simulink library "rappid_564xl_ec_toolbox"  (Simulink 8.1)
settings: Solver=FixedStepDiscrete  StartTime=0.0  StopTime=10.0  RelTol=1e-3
undefined symbols (not defined in the file or in its folder): CTU_unit, mem_AddrLW, mem_AddrUP, rappid_564xl_adc_input_support_rev2, rappid_564xl_can_support_rev2, read_mem_AddrLW, read_mem_AddrUP
(part 2 of 5)

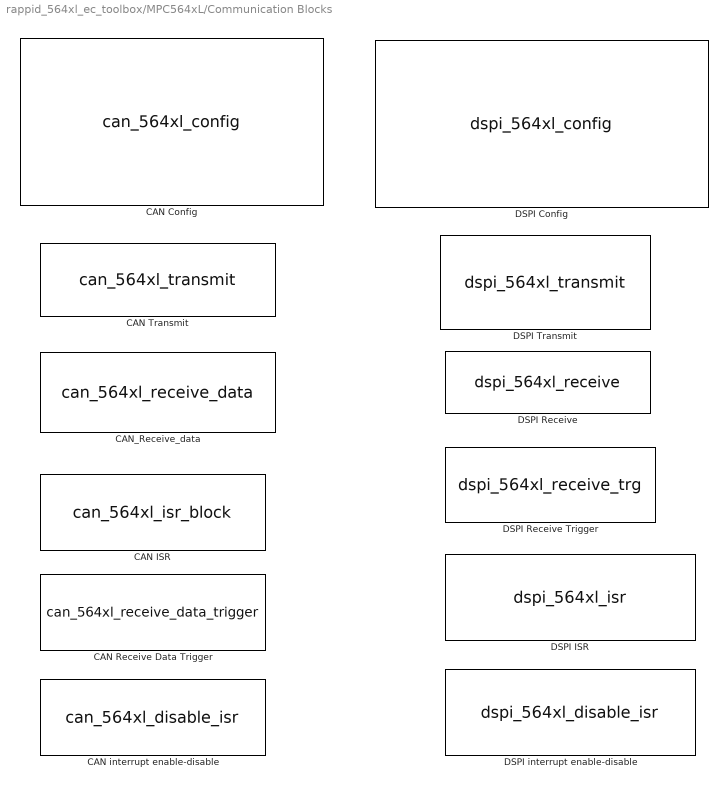
== system rappid_564xl_ec_toolbox/MPC564xL/Communication Blocks ==
  CAN Config : S-Function  Priority=1  LoadFcn=rappid_564xl_can_support_rev2(gcb);  FunctionName=can_564xl_config  Parameters=can_unit_v2, MCR, CTRL  EnableBusSupport=off  mask(flexcan_564xl_config_block){can_unit=A, can_unit_v2=0, can_idam=A - One full ID (standard or extended) per filter element., can_srx_dis=1 - Self reception disabled, can_presdiv=4, can_rjw=3, can_pseg1=3, can_pseg2=3, can_clk_src=0 - The CAN engine clock source is the oscillator clock, can_lpb=0 - Loop Back disabled, can_smp=1 - Three samples are used to determine the value of the received bit, can_boff_rec=0 - Automatic recovering from Bus Off state enabled, can_tsyn=0 - Timer Sync feature disabled, can_lbuf=0 - Buffer with highest priority is transmitted first, can_lom=0 - Listen Only Mode is deactivated, can_propseg=6}
      mask prompts: can_unit "CAN Bus"; can_unit_v2 "CAN Bus"; can_idam "ID Acceptance Mode"; can_srx_dis "Self Reception Disable"; can_presdiv "Prescaler Divider (0-255)"; can_rjw "Resync Jump Width"; can_pseg1 "Phase Segment 1"; can_pseg2 "Phase Segment 2"; can_clk_src "CAN Engine Clock Source"; can_lpb "Loop Back"; can_smp "Sampling Mode"; can_boff_rec "Bus Off Recovery Mode"; can_tsyn "Timer Sync Mode"; can_lbuf "Lowest Buffer Transmitted First"; can_lom "Listen-Only Mode"; can_propseg "Propagation Segment"
      mask help: This block allows to configure the FlexCan module.
      mask init:
      | crlf = sprintf('\n');
      | 
      | canUnit     = num2str(get_param(gcb,'can_unit_v2'));
      | canIDAM     = get_param(gcb,'can_idam');
      | 
      | MCR = 1342177343;
      | if (strcmp(canIDAM,'A - One full ID (standard or extended) per filter element.'))
      |     canIDAM = 'A - One full ID ';
      | elseif (strcmp(canIDAM,'B - Two full standard IDs or two partial 14-bit extended IDs per filter element.'))
      |     canIDAM = 'B - Two full standard IDs';
      |     MCR = bitset(uint32(MCR), 32-23);
      | elseif (strcmp(canIDAM,'C - Four partial 8-bit IDs (standard or extended) per filter element.'))
      |     canIDAM = 'C - Four partial 8-bit IDs';
      |     MCR = bitset(uint32(MCR), 32-22);
      | elseif (strcmp(canIDAM,'D - All frames rejected.'))
      |     canIDAM = 'Rejected';
      |     MCR = bitset(uint32(MCR), 32-23);
      |     MCR = bitset(uint32(MCR), 32-22);
      | end
      | 
      | if ( strcmp( num2str(get_param(gcb,'can_srx_dis')), 'on'))
      |     MCR = bitset(uint32(MCR), 32-14);
      | end
      | 
      | CTRL = 0;
      | 
      | CTRL = bitshift(uint32(str2num(get_param(gcb, 'can_presdiv'))),31-7);
      | CTRL = bitor( CTRL, bitshift(uint32(str2num(get_param(gcb, 'can_rjw'))),31-9));
      | CTRL = bitor( CTRL, bitshift(uint32(str2num(get_param(gcb, 'can_pseg1'))),31-12));
      | CTRL = bitor( CTRL, bitshift(uint32(str2num(get_param(gcb, 'can_pseg2'))),31-15));
      | 
      | if ( strcmp( get_param(gcb,'can_clk_src'), '1 - The CAN engine clock source is the bus clock'))
      |     CTRL = bitset(uint32(CTRL), 32-18);
      | end
      | 
      | if ( strcmp( get_param(gcb,'can_lpb'), '1 - Loop Back enabled'))
      |     CTRL = bitset(uint32(CTRL), 32-19);
      | end
      | 
      | if ( strcmp( get_param(gcb,'can_smp'), '1 - Three samples are used to determine the value of the received bit'))
      |     CTRL = bitset(uint32(CTRL), 32-24);
      | end
      | 
      | if ( strcmp( get_param(gcb,'can_boff_rec'), '1 - Automatic recovering from Bus Off state disabled'))
      |     CTRL = bitset(uint32(CTRL), 32-25);
      | end
      | 
      | if ( strcmp( get_param(gcb,'can_tsyn'), '1 - Timer Sync feature enabled'))
      |     CTRL = bitset(uint32(CTRL), 32-26);
      | end
      | 
      | if ( strcmp( get_param(gcb,'can_lbuf'), '1 - Lowest number buffer is transmitted first'))
      |     CTRL = bitset(uint32(CTRL), 32-27);
      | end
      | 
      | if ( strcmp( get_param(gcb,'can_lom'), '1 - FlexCAN module operates in Listen Only Mode'))
      |     CTRL = bitset(uint32(CTRL), 32-28);
      | end
      | 
      | CTRL = bitor( CTRL, bitshift(uint32(str2num(get_param(gcb, 'can_propseg'))),31-31));
      | 
      | maskStr = [ 'CAN Bus ',canUnit, crlf,...
      |     'ID Acceptance Mode ', canIDAM,...
      |     ];
      | 
      | if strcmp(canUnit ,'0')
      |    value_new = 'A';
      | else                                     
      |    value_new = 'B';         
      | end                                                                               
      | set_param(gcb, 'can_unit', value_new);
      mask Help: web([rappid_block_help,filesep,'CAN_config.htm']);
      mask TypeOptions can_unit: A | B
      mask TypeOptions can_unit_v2: 0 | 1
      mask TypeOptions can_idam: A - One full ID (standard or extended) per filter element. | B - Two full standard IDs or two partial 14-bit extended IDs per filter element. | C - Four partial 8-bit IDs (standard or extended) per filter element. | D - All frames rejected.
      mask TypeOptions can_srx_dis: 0 - Self reception enabled | 1 - Self reception disabled
      mask TypeOptions can_rjw: 0 | 1 | 2 | 3
      mask TypeOptions can_pseg1: 0 | 1 | 2 | 3 | 4 | 5 | 6 | 7
      mask TypeOptions can_pseg2: 1 | 2 | 3 | 4 | 5 | 6 | 7
      mask TypeOptions can_clk_src: 0 - The CAN engine clock source is the oscillator clock | 1 - The CAN engine clock source is the bus clock
      mask TypeOptions can_lpb: 0 - Loop Back disabled | 1 - Loop Back enabled
      mask TypeOptions can_smp: 0 - One sample is used to determine the bit value | 1 - Three samples are used to determine the value of the received bit
      mask TypeOptions can_boff_rec: 0 - Automatic recovering from Bus Off state enabled | 1 - Automatic recovering from Bus Off state disabled
      mask TypeOptions can_tsyn: 0 - Timer Sync feature disabled | 1 - Timer Sync feature enabled
      mask TypeOptions can_lbuf: 0 - Buffer with highest priority is transmitted first | 1 - Lowest number buffer is transmitted first
      mask TypeOptions can_lom: 0 - Listen Only Mode is deactivated | 1 - FlexCAN module operates in Listen Only Mode
      mask TypeOptions can_propseg: 0 | 1 | 2 | 3 | 4 | 5 | 6 | 7
      mask Display: disp(maskStr)
  CAN ISR : S-Function  LoadFcn=rappid_564xl_can_support_rev2(gcb);  FunctionName=can_564xl_isr_block  Parameters=can_unit_v2, can_isr_prio, canMode, canFlags  EnableBusSupport=off  mask(flexcan_564xl_isr_block){can_unit=A, can_unit_v2=0, can_isr_prio=1, can_isr_mode=Errors, can_wrn_tx=on, can_wrn_rx=on}
      mask prompts: can_unit "CAN Bus"; can_unit_v2 "CAN Bus"; can_isr_prio "ISR Priority"; can_isr_mode "Can ISR"; can_wrn_tx "Tx Warning Interrupt"; can_wrn_rx "Rx Warning Interrupt"
      mask help: This block allows user to process FlexCan ISR's
      mask init:
      | crlf = sprintf('\n');
      | 
      | canUnit     = num2str(get_param(gcb,'can_unit_v2'));
      | canISRPrio  = num2str(get_param(gcb,'can_isr_prio'));
      | canISRMode  = get_param(gcb, 'can_isr_mode');
      | canTxWrn    = get_param(gcb, 'can_wrn_tx');
      | canRxWrn    = get_param(gcb, 'can_wrn_rx');
      | 
      | canMode = 0;
      | TxWrn = 0;
      | RxWrn = 0;
      | 
      | maskStr = [ 'CAN Bus ',canUnit, crlf, 'ISR Priority ',canISRPrio, crlf,...
      |         'CAN ISR Mode ',canISRMode, crlf];
      |              
      | if (strcmp(canISRMode,'Warnings'))
      |     maskStr = [ maskStr, 'TxWarning ', canTxWrn, crlf, 'RxWarning' canRxWrn];
      |     
      |     canMode = 1;
      |     
      |     if (strcmp(canTxWrn,'on'))
      |         TxWrn = 1;
      |     end
      |     if (strcmp(canRxWrn,'on'))
      |         RxWrn = 1;
      |     end
      |    
      |     
      | end
      | canFlags =[TxWrn, RxWrn]; 
      | 
      | if strcmp(canUnit ,'0')
      |    value_new = 'A';
      | else                                     
      |    value_new = 'B';         
      | end                                                                               
      | set_param(gcb, 'can_unit', value_new);
      mask Help: web([rappid_block_help,filesep,'CAN_isr.htm']);
      mask TypeOptions can_unit: A | B
      mask TypeOptions can_unit_v2: 0 | 1
      mask TypeOptions can_isr_prio: 1 | 2 | 3 | 4 | 5 | 6 | 7 | 8 | 9 | 10 | 11 | 12 | 13 | 14 | 15
      mask TypeOptions can_isr_mode: Errors | Warnings
      mask Callback can_isr_mode:
      | maskVis = get_param(gcb, 'MaskVisibilities');
      | 
      | if (strcmp (get_param(gcb, 'can_isr_mode'), 'Errors'))
      |     maskVis{5} = 'off';
      |     maskVis{6} = 'off';
      | else
      |     maskVis{5} = 'on';
      |     maskVis{6} = 'on';
      | end
      | 
      | set_param(gcb,'MaskVisibilities', maskVis);
      mask Display:
      | disp(maskStr)
      | port_label('output', 1, 'Trigger');
      | port_label('output', 2, 'Mask');
  CAN Receive Data Trigger : S-Function  LoadFcn=rappid_564xl_can_support_rev2(gcb);  FunctionName=can_564xl_receive_data_trigger  Parameters=can_unit_v2, can_buffer, can_id  EnableBusSupport=off  mask(flexcan_564xl_receive_data_trigger_block){can_unit=A, can_unit_v2=0, can_buffer=0, can_id=0, can_isr_prio=0}
      mask prompts: can_unit "CAN Bus"; can_unit_v2 "CAN Bus"; can_buffer "Buffer (0 to 31)"; can_id "ID"; can_isr_prio "ISR Priority"
      mask help: This block allows user to receive data through CAN interface
      mask init:
      | crlf = sprintf('\n');
      | 
      | canUnit     = num2str(get_param(gcb,'can_unit_v2'));
      | canBuffer   = num2str(get_param(gcb,'can_buffer'));
      | canID       = num2str(get_param(gcb,'can_id'));
      | canISRPrio  = num2str(get_param(gcb,'can_isr_prio'));
      | maskStr = [ 'CAN Bus ',canUnit, crlf,'CAN Buffer ', canBuffer, crlf...
      |     'CAN Message ID ', canID, crlf, 'CAN ISR Priority ', canISRPrio ];
      | 
      | if strcmp(canUnit ,'0')
      |    value_new = 'A';
      | else                                     
      |    value_new = 'B';         
      | end                                                                               
      | set_param(gcb, 'can_unit', value_new);
      mask Help: web([rappid_block_help,filesep,'CAN_receive_trigger.htm']);
      mask TypeOptions can_unit: A | B
      mask TypeOptions can_unit_v2: 0 | 1
      mask TypeOptions can_buffer: 0 | 1 | 2 | 3 | 4 | 5 | 6 | 7 | 8 | 9 | 10 | 11 | 12 | 13 | 14 | 15 | 16 | 17 | 18 | 19 | 20 | 21 | 22 | 23 | 24 | 25 | 26 | 27 | 28 | 29 | 30 | 31
      mask TypeOptions can_isr_prio: 0 | 1 | 2 | 3 | 4 | 5 | 6 | 7 | 8 | 9 | 10 | 11 | 12 | 13 | 14 | 15
      mask Display:
      | disp(maskStr)
      | port_label('output', 1, 'Trigger');
      | port_label('output', 2, 'ID');
      | port_label('output', 3, 'ID Type');
      | port_label('output', 4, 'Message');
      | port_label('output', 5, 'Time stamp');
  CAN Transmit : S-Function  LoadFcn=rappid_564xl_can_support_rev2(gcb);  FunctionName=can_564xl_transmit  Parameters=can_unit_v2, can_buffer, can_id  EnableBusSupport=off  mask(flexcan_564xl_transmit_block){can_unit=A, can_unit_v2=0, can_buffer=0, can_id=0}
      mask prompts: can_unit "CAN Bus"; can_unit_v2 "CAN Bus"; can_buffer "Buffer (0 to 31)"; can_id "ID"
      mask help: This block allows user to transmit data throught CAN interface.
      mask init:
      | crlf = sprintf('\n');
      | 
      | canUnit     = num2str(get_param(gcb,'can_unit_v2'));
      | canBuffer   = num2str(get_param(gcb,'can_buffer'));
      | canID       = num2str(get_param(gcb,'can_id'));
      | maskStr = [ 'CAN Bus ',canUnit, crlf,'CAN Buffer ', canBuffer, crlf...
      |     'CAN Message ID ', canID];
      | 
      | if strcmp(canUnit ,'0')
      |    value_new = 'A';
      | else                                     
      |    value_new = 'B';         
      | end                                                                               
      | set_param(gcb, 'can_unit', value_new);
      mask Help: web([rappid_block_help,filesep,'CAN_transmit.htm']);
      mask TypeOptions can_unit: A | B
      mask TypeOptions can_unit_v2: 0 | 1
      mask TypeOptions can_buffer: 0 | 1 | 2 | 3 | 4 | 5 | 6 | 7 | 8 | 9 | 10 | 11 | 12 | 13 | 14 | 15 | 16 | 17 | 18 | 19 | 20 | 21 | 22 | 23 | 24 | 25 | 26 | 27 | 28 | 29 | 30 | 31
      mask Display:
      | disp(maskStr)
      | port_label('input', 1, 'Message');
      | port_label('input', 2, 'Lenght');
  CAN interrupt enable-disable : S-Function  FunctionName=can_564xl_disable_isr  Parameters="can_unit,   canFlags"  EnableBusSupport=off  mask(flexcan_564xl_isr_enable){can_unit=0, can_err_enable=off, can_wrn_tx=off, can_wrn_rx=off}
      mask prompts: can_unit "CAN Bus"; can_err_enable "Enable Error Interrupt"; can_wrn_tx "Enable Tx Warning Interrupt"; can_wrn_rx "Enable Rx Warning Interrupt"
      mask help: This block enables or disables the interrupt for each PIT block.
      mask init:
      | crlf = sprintf('\n');
      | 
      | canUnit     = num2str(get_param(gcb,'can_unit'));
      | canErr      = get_param(gcb, 'can_err_enable');
      | canTxWrn    = get_param(gcb, 'can_wrn_tx');
      | canRxWrn    = get_param(gcb, 'can_wrn_rx');
      | 
      | maskStr = [ 'CAN Bus: ', canUnit, crlf, 'Error interrupt: ', canErr, crlf, 'TX Warning interrupt: ', canTxWrn, crlf,'RX Warning interrupt: ', canRxWrn]; 
      | 
      | ErrInt = 0;
      | TxWrn = 0;
      | RxWrn = 0;
      | 
      | if (strcmp(canTxWrn,'on'))
      |     TxWrn = 1;
      | end
      | if (strcmp(canRxWrn,'on'))
      |     RxWrn = 1;
      | end
      | if (strcmp(canErr,'on'))
      |     ErrInt = 1;
      | end
      |      
      | canFlags =[TxWrn, RxWrn, ErrInt];
      mask Help: web([rappid_block_help,filesep,'CAN_isr_enable.htm']);
      mask TypeOptions can_unit: 0 | 1
      mask Display: disp(maskStr)
  CAN_Receive_data : S-Function  LoadFcn=rappid_564xl_can_support_rev2(gcb);  FunctionName=can_564xl_receive_data  Parameters=can_unit_v2, can_buffer, can_id  EnableBusSupport=off  mask(flexcan_564xl_receive_data_block){can_unit=A, can_unit_v2=0, can_buffer=0, can_id=0}
      mask prompts: can_unit "CAN Bus"; can_unit_v2 "CAN Bus"; can_buffer "Buffer (0 to 31)"; can_id "ID"
      mask help: This block allows user to receive data through CAN interface
      mask init:
      | crlf = sprintf('\n');
      | 
      | canUnit     = num2str(get_param(gcb,'can_unit_v2'));
      | canBuffer   = num2str(get_param(gcb,'can_buffer'));
      | canID       = num2str(get_param(gcb,'can_id'));
      | maskStr = [ 'CAN Bus ',canUnit, crlf,'CAN Buffer ', canBuffer, crlf...
      |     'CAN Message ID ', canID ];
      | 
      | if strcmp(canUnit ,'0')
      |    value_new = 'A';
      | else                                     
      |    value_new = 'B';         
      | end                                                                               
      | set_param(gcb, 'can_unit', value_new);
      | 
      | clear value_new;
      mask Help: web([rappid_block_help,filesep,'CAN_receive.htm']);
      mask TypeOptions can_unit: A | B
      mask TypeOptions can_unit_v2: 0 | 1
      mask TypeOptions can_buffer: 0 | 1 | 2 | 3 | 4 | 5 | 6 | 7 | 8 | 9 | 10 | 11 | 12 | 13 | 14 | 15 | 16 | 17 | 18 | 19 | 20 | 21 | 22 | 23 | 24 | 25 | 26 | 27 | 28 | 29 | 30 | 31
      mask Display:
      | disp(maskStr)
      | port_label('output', 1, 'ID');
      | port_label('output', 2, 'ID Type');
      | port_label('output', 3, 'Message');
      | port_label('output', 4, 'Time stamp');
  DSPI Config : S-Function  Priority=1  FunctionName=dspi_564xl_config  Parameters=dspiNum, MCR, CTAR  EnableBusSupport=off  mask(DSPI_564xL_Config){dspi_Num=0, dspi_Mode=Master, dspi_MTFE=off, dspi_CONT_SCKE=off, dspi_PCSSE=off, dspi_ROOE=off, dspi_DIS_TXF=Disable, dspi_DIS_RXF_v2=Disable, dspi_SMPL_PT=DSPI samples SIN at driving SCK edge, dspi_FMSZ=16, dspi_CPOL=Low, dspi_CPHA=Data is captured on the leading edge of SCK and changed on the following edge, dspi_LSBFE=MSB first, dspi_DBR=off, dspi_PCSSCK=1, dspi_PASC=1, dspi_PDT=5, dspi_PBR=5, dspi_CSSCK=256, dspi_ASC=256, dspi_DT=8, dspi_BR=128, dspi_PCSIS0=High, dspi_PCSIS1=High, dspi_PCSIS2=High, dspi_PCSIS3=High, dspi_PCSIS4=High, dspi_PCSIS5=High, dspi_PCSIS6=High, dspi_PCSIS7=High, dspi_DIS_RXF=Oops}
      mask prompts: dspi_Num "DSPI"; dspi_Mode "Mode"; dspi_MTFE "Modified Timing Format Enabled"; dspi_CONT_SCKE "Continuous SCK"; dspi_PCSSE "Chip Selectr Strobe Enable"; dspi_ROOE "Receive FIFO Overflow Overwrite Enable"; dspi_DIS_TXF "Transmit FIFO"; dspi_DIS_RXF_v2 "Receive FIFO"; dspi_SMPL_PT "Sample Point"; dspi_FMSZ "Frame Size"; dspi_CPOL "Clock Polarity"; dspi_CPHA "Clock Phase"; dspi_LSBFE "Data Transfer Mode"; dspi_DBR "Double Baud Rate (DBR)"; dspi_PCSSCK "PCS to SCK Delay Prescaler (PCSSCK)"; dspi_PASC "After SCK Delay Prescaler (PASC)"; dspi_PDT "Delay After Transfer Prescaler (PDT)"; dspi_PBR "Baud Rate Prescaler (PBR)"; dspi_CSSCK "PCS to SCK Delay Scaler (CSSCK)"; dspi_ASC "After SCK delay Scaler (ASC)"; dspi_DT "Delay after Transfer Scaler (DT)"; dspi_BR "Baud Rate Scaler (BR)"; dspi_PCSIS0 "Chip Select Inactive State 0"; dspi_PCSIS1 "Chip Select Inactive State 1"; dspi_PCSIS2 "Chip Select Inactive State 2"; dspi_PCSIS3 "Chip Select Inactive State 3"; dspi_PCSIS4 "Chip Select Inactive State 4"; dspi_PCSIS5 "Chip Select Inactive State 5"; dspi_PCSIS6 "Chip Select Inactive State 6"; dspi_PCSIS7 "Chip Select Inactive State 7"; dspi_DIS_RXF "Receive FIFO"
      mask help: Configure DSPI Block
      mask init:
      | crlf = sprintf('\n');
      | 
      | dspiNum = get_param(gcb, 'dspi_Num');
      | dspiMode = get_param(gcb, 'dspi_Mode');
      | dspiMTFE = get_param(gcb, 'dspi_MTFE');
      | dspiPCSSE = get_param(gcb, 'dspi_PCSSE');
      | dspiROOE = get_param(gcb, 'dspi_ROOE');
      | 
      | dspiDISTXF = get_param(gcb, 'dspi_DIS_TXF');
      | dspiDISRXF = get_param(gcb, 'dspi_DIS_RXF_v2');
      | 
      | dspiSMPLPT = get_param(gcb, 'dspi_SMPL_PT');
      | 
      | st = ['DSPI: ', dspiNum, crlf, 'Mode: ', dspiMode, crlf...
      |     'Modified Timing Format: ', dspiMTFE, crlf...
      |     'Peripheral Chip Select Strobe Enable: ', dspiPCSSE, crlf,...
      |     'Receive Owerwrite: ', dspiROOE, crlf,...
      |     'Transmit FIFO: ', dspiDISTXF, crlf, ...
      |     'Receive FIFO: ', dspiDISRXF, crlf, ...
      |     'Sampling Point: ', dspiSMPLPT];
      | 
      | dspiNum = str2num(dspiNum);
      | 
      | MCR = 1;
      | 
      | if ( strcmp(dspiMode,'Master'))
      |     MCR = bitset(uint32(MCR),32);
      | else
      |     MCR = bitset(uint32(MCR),32, 0);
      | end
      | 
      | if ( strcmp(get_param(gcb, 'dspi_CONT_SCKE'),'on'))
      |     MCR = bitset(uint32(MCR),31);
      | else
      |     MCR = bitset(uint32(MCR),31, 0);
      | end
      | 
      | if ( strcmp(dspiMTFE, 'on'))
      |    MCR = bitset(uint32(MCR),27);
      | else
      |     MCR = bitset(uint32(MCR), 27, 0);
      | end  
      | 
      | if ( strcmp(dspiPCSSE, 'on'))
      |    MCR = bitset(uint32(MCR),26);
      | else
      |     MCR = bitset(uint32(MCR), 26, 0);
      | end 
      |     
      | if ( strcmp(dspiROOE, 'on'))
      |    MCR = bitset(uint32(MCR),25);
      | else
      |     MCR = bitset(uint32(MCR), 25, 0);
      | end
      | 
      | if ( strcmp(get_param(gcb, 'dspi_PCSIS7'),'High' ))
      |     MCR = bitset(uint32(MCR), 24);
      | else
      |     MCR = bitset(uint32(MCR), 24, 0);
      | end
      | 
      | if ( strcmp(get_param(gcb, 'dspi_PCSIS6'),'High' ))
      |     MCR = bitset(uint32(MCR), 23);
      | else
      |     MCR = bitset(uint32(MCR), 23, 0);
      | end
      | 
      | if ( strcmp(get_param(gcb, 'dspi_PCSIS5'),'High' ))
      |     MCR = bitset(uint32(MCR), 22);
      | else
      |     MCR = bitset(uint32(MCR), 22, 0);
      | end
      | 
      | if ( strcmp(get_param(gcb, 'dspi_PCSIS4'),'High' ))
      |     MCR = bitset(uint32(MCR), 21);
      | else
      |     MCR = bitset(uint32(MCR), 21, 0);
      | end
      | 
      | if ( strcmp(get_param(gcb, 'dspi_PCSIS3'),'High' ))
      |     MCR = bitset(uint32(MCR), 20);
      | else
      |     MCR = bitset(uint32(MCR), 20, 0);
      | end
      | 
      | if ( strcmp(get_param(gcb, 'dspi_PCSIS2'),'High' ))
      |     MCR = bitset(uint32(MCR), 19);
      | else
      |     MCR = bitset(uint32(MCR), 19, 0);
      | end
      | 
      | if ( strcmp(get_param(gcb, 'dspi_PCSIS1'),'High' ))
      |     MCR = bitset(uint32(MCR), 18);
      | else
      |     MCR = bitset(uint32(MCR), 18, 0);
      | end
      | 
      | if ( strcmp(get_param(gcb, 'dspi_PCSIS0'),'High' ))
      |     MCR = bitset(uint32(MCR), 17);
      | else
      |     MCR = bitset(uint32(MCR), 17, 0);
      | end
      | 
      | if ( strcmp(get_param(gcb, 'dspi_DIS_TXF'),'Enable'))
      |     MCR = bitset(uint32(MCR), 14, 0);
      | else
      |     MCR = bitset(uint32(MCR), 14);
      | end
      | 
      | if ( strcmp(get_param(gcb, 'dspi_DIS_RXF'),'Enable'))
      |     MCR = bitset(uint32(MCR), 13, 0);
      | else
      |     MCR = bitset(uint32(MCR), 13);
      | end
      | 
      | if ( strcmp(get_param(gcb, 'dspi_SMPL_PT'),'DSPI samples SIN at driving SCK edge'))
      |     MCR = bitset(uint32(MCR), 10, 0);
      |     MCR = bitset(uint32(MCR), 9, 0);
      | elseif (strcmp(get_param(gcb, 'dspi_SMPL_PT'),'DSPI samples SIN one system clock after driving SCK edge'))
      |     MCR = bitset(uint32(MCR), 10, 0);
      |     MCR = bitset(uint32(MCR), 9);
      | else
      |     MCR = bitset(uint32(MCR), 10);
      |     MCR = bitset(uint32(MCR), 9, 0);
      | end
      | 
      | 
      | CTAR = 0;
      | 
      | if ( strcmp(get_param(gcb, 'dspi_DBR'), 'on'))
      |     CTAR = bitset(uint32(CTAR), 32);
      | else    
      |     CTAR = bitset(uint32(CTAR), 32, 0);
      | end
      |       
      | temp = 0;
      | temp = str2num(get_param(gcb, 'dspi_FMSZ'));
      | temp = temp - 1;
      | temp = bitshift(uint32(temp),27);
      | CTAR = bitor( uint32(CTAR), uint32(temp));
      | 
      | if (strcmp( get_param(gcb, 'dspi_CPOL'), 'Low'))
      |     CTAR = bitset( uint32(CTAR), 27, 0);
      | else
      |     CTAR = bitset( uint32(CTAR), 27);
      | end
      | 
      | 
      | if (strcmp( get_param(gcb, 'dspi_CPHA'), 'Data is captured on the leading edge of SCK and changed on the following edge'))
      |     CTAR = bitset( uint32(CTAR), 26, 0);
      | else
      |     CTAR = bitset( uint32(CTAR), 26);
      | end
      | 
      | if (strcmp( get_param(gcb, 'dspi_LSBFE'), 'MSB first'))
      |     CTAR = bitset( uint32(CTAR), 25, 0);
      | else
      |     CTAR = bitset( uint32(CTAR), 25);
      | end
      | 
      | temp = str2num( get_param(gcb, 'dspi_PCSSCK'));
      | temp = bitshift(uint8(temp), -1);
      | temp = bitshift(uint32(temp), 22);
      | CTAR = bitor(uint32(CTAR), temp);
      | 
      | temp = str2num( get_param(gcb, 'dspi_PASC'));
      | temp = bitshift(uint8(temp), -1);
      | temp = bitshift(uint32(temp), 20);
      | CTAR = bitor(uint32(CTAR), temp);
      | 
      | temp = str2num( get_param(gcb, 'dspi_PDT'));
      | temp = bitshift(uint8(temp), -1);
      | temp = bitshift(uint32(temp), 18);
      | CTAR = bitor(uint32(CTAR), temp);
      | 
      | temp = str2num( get_param(gcb, 'dspi_PBR'));
      | temp = bitshift(uint8(temp), -1);
      | temp = bitshift(uint32(temp), 16);
      | CTAR = bitor(uint32(CTAR), temp);
      | 
      | 
      | i = str2num('12');
      | temp = str2num( get_param(gcb, 'dspi_CSSCK'));
      | if (temp == 2)
      |      CTAR = bitor(uint32(CTAR), bitshift(uint32(0),i));
      | elseif (temp == 4)
      |     CTAR = bitor(uint32(CTAR), bitshift(uint32(1),i));
      | elseif (temp == 8)
      |     CTAR = bitor(uint32(CTAR), bitshift(uint32(2),i));
      | elseif (temp == 16)
      |     CTAR = bitor(uint32(CTAR), bitshift(uint32(3),i));
      | elseif (temp == 32)
      |     CTAR = bitor(uint32(CTAR), bitshift(uint32(4),i));
      | elseif (temp == 64)
      |     CTAR = bitor(uint32(CTAR), bitshift(uint32(5),i));
      | elseif (temp == 128)
      |     CTAR = bitor(uint32(CTAR), bitshift(uint32(6),i));
      | elseif (temp == 256)
      |     CTAR = bitor(uint32(CTAR), bitshift(uint32(7),i));
      | elseif (temp == 512)
      |     CTAR = bitor(uint32(CTAR), bitshift(uint32(8),i));
      | elseif (temp == 1024)
      |     CTAR = bitor(uint32(CTAR), bitshift(uint32(9),i));
      | elseif (temp == 2048)
      |     CTAR = bitor(uint32(CTAR), bitshift(uint32(10),i));
      | elseif (temp == 4096)
      |     CTAR = bitor(uint32(CTAR), bitshift(uint32(11),i));
      | elseif (temp == 8192)
      |     CTAR = bitor(uint32(CTAR), bitshift(uint32(12),i));
      | elseif (temp == 16384)
      |     CTAR = bitor(uint32(CTAR), bitshift(uint32(13),i));
      | elseif (temp == 32768)
      |     CTAR = bitor(uint32(CTAR), bitshift(uint32(14),i));
      | elseif (temp == 65536)
      |     CTAR = bitor(uint32(CTAR), bitshift(uint32(15),i));
      | end	
      | 	
      | 	
      | i=str2num('8');
      | temp = str2num( get_param(gcb, 'dspi_ASC'));
      | if (temp == 2)
      |     CTAR = bitor(uint32(CTAR), bitshift(0,i));
      | elseif (temp == 4)
      |     CTAR = bitor(uint32(CTAR), bitshift(1,i));
      | elseif (temp == 8)
      |     CTAR = bitor(uint32(CTAR), bitshift(2,i));
      | elseif (temp == 16)
      |     CTAR = bitor(uint32(CTAR), bitshift(3,i));
      | elseif (temp == 32)
      |     CTAR = bitor(uint32(CTAR), bitshift(4,i));
      | elseif (temp == 64)
      |     CTAR = bitor(uint32(CTAR), bitshift(5,i));
      | elseif (temp == 128)
      |     CTAR = bitor(uint32(CTAR), bitshift(6,i));
      | elseif (temp == 256)
      |     CTAR = bitor(uint32(CTAR), bitshift(7,i));
      | elseif (temp == 512)
      |     CTAR = bitor(uint32(CTAR), bitshift(8,i));
      | elseif (temp == 1024)
      |     CTAR = bitor(uint32(CTAR), bitshift(9,i));
      | elseif (temp == 2048)
      |     CTAR = bitor(uint32(CTAR), bitshift(10,i));
      | elseif (temp == 4096)
      |     CTAR = bitor(uint32(CTAR), bitshift(11,i));
      | elseif (temp == 8192)
      |     CTAR = bitor(uint32(CTAR), bitshift(12,i));
      | elseif (temp == 16384)
      |     CTAR = bitor(uint32(CTAR), bitshift(13,i));
      | elseif (temp == 32768)
      |     CTAR = bitor(uint32(CTAR), bitshift(14,i));
      | elseif (temp == 65536)
      |     CTAR = bitor(uint32(CTAR), bitshift(15,i));
      | end
      | 
      | i=str2num('4');
      | temp = str2num( get_param(gcb, 'dspi_DT'));
      | if (temp == 2)
      |     CTAR = bitor(uint32(CTAR), bitshift(0,i));
      | elseif (temp == 4)
      |     CTAR = bitor(uint32(CTAR), bitshift(1,i));
      | elseif (temp == 8)
      |     CTAR = bitor(uint32(CTAR), bitshift(2,i));
      | elseif (temp == 16)
      |     CTAR = bitor(uint32(CTAR), bitshift(3,i));
      | elseif (temp == 32)
      |     CTAR = bitor(uint32(CTAR), bitshift(4,i));
      | elseif (temp == 64)
      |     CTAR = bitor(uint32(CTAR), bitshift(5,i));
      | elseif (temp == 128)
      |     CTAR = bitor(uint32(CTAR), bitshift(6,i));
      | elseif (temp == 256)
      |     CTAR = bitor(uint32(CTAR), bitshift(7,i));
      | elseif (temp == 512)
      |     CTAR = bitor(uint32(CTAR), bitshift(8,i));
      | elseif (temp == 1024)
      |     CTAR = bitor(uint32(CTAR), bitshift(9,i));
      | elseif (temp == 2048)
      |     CTAR = bitor(uint32(CTAR), bitshift(10,i));
      | elseif (temp == 4096)
      |     CTAR = bitor(uint32(CTAR), bitshift(11,i));
      | elseif (temp == 8192)
      |     CTAR = bitor(uint32(CTAR), bitshift(12,i));
      | elseif (temp == 16384)
      |     CTAR = bitor(uint32(CTAR), bitshift(13,i));
      | elseif (temp == 32768)
      |     CTAR = bitor(uint32(CTAR), bitshift(14,i));
      | elseif (temp == 65536)
      |     CTAR = bitor(uint32(CTAR), bitshift(15,i));
      | end
      | 
      | 
      | i=str2num('0');
      | temp = str2num( get_param(gcb, 'dspi_BR'));
      | if (temp == 2)
      |     CTAR = bitor(uint32(CTAR), bitshift(0,i));
      | elseif (temp == 4)
      |     CTAR = bitor(uint32(CTAR), bitshift(1,i));
      | elseif (temp == 6)
      |     CTAR = bitor(uint32(CTAR), bitshift(2,i));
      | elseif (temp == 8)
      |     CTAR = bitor(uint32(CTAR), bitshift(3,i));
      | elseif (temp == 16)
      |     CTAR = bitor(uint32(CTAR), bitshift(4,i));
      | elseif (temp == 32)
      |     CTAR = bitor(uint32(CTAR), bitshift(5,i));
      | elseif (temp == 64)
      |     CTAR = bitor(uint32(CTAR), bitshift(6,i));
      | elseif (temp == 128)
      |     CTAR = bitor(uint32(CTAR), bitshift(7,i));
      | elseif (temp == 256)
      |     CTAR = bitor(uint32(CTAR), bitshift(8,i));
      | elseif (temp == 512)
      |     CTAR = bitor(uint32(CTAR), bitshift(9,i));
      | elseif (temp == 1024)
      |     CTAR = bitor(uint32(CTAR), bitshift(10,i));
      | elseif (temp == 2048)
      |     CTAR = bitor(uint32(CTAR), bitshift(11,i));
      | elseif (temp == 4096)
      |     CTAR = bitor(uint32(CTAR), bitshift(12,i));
      | elseif (temp == 8192)
      |     CTAR = bitor(uint32(CTAR), bitshift(13,i));
      | elseif (temp == 16384)
      |     CTAR = bitor(uint32(CTAR), bitshift(14,i));
      | elseif (temp == 32768)
      |     CTAR = bitor(uint32(CTAR), bitshift(15,i));
      | end
      mask Help: web([rappid_block_help,filesep,'DSPI_Config.htm']);
      mask TypeOptions dspi_Num: 0 | 1 | 2
      mask TypeOptions dspi_Mode: Master | Slave
      mask Callback dspi_Mode:
      | MaskEnables = get_param(gcb, 'MaskEnables');
      | Mode = get_param(gcb, 'dspi_Mode');
      | 
      | if(strcmp(Mode, 'Master'))
      |     for i = 3:30
      |         MaskEnables{i} = 'on';
      |     end
      | else
      |     for i = 3:30
      |         MaskEnables{i} = 'off';
      |     end
      | 
      |     MaskEnables{10} = 'on'; %%frame size
      |     MaskEnables{11} = 'on';
      |     MaskEnables{12} = 'on';
      | end
      | 
      | set_param(gcb, 'MaskEnables', MaskEnables);
      mask TypeOptions dspi_DIS_TXF: Enable | Disable
      mask TypeOptions dspi_DIS_RXF_v2: Enable | Disable
      mask TypeOptions dspi_SMPL_PT: DSPI samples SIN at driving SCK edge | DSPI samples SIN one system clock after driving SCK edge | DSPI samples SIN two system clocks after driving SCK edge
      mask TypeOptions dspi_FMSZ: 3 | 4 | 5 | 6 | 7 | 8 | 9 | 10 | 11 | 12 | 13 | 14 | 15 | 16
      mask TypeOptions dspi_CPOL: Low | High
      mask TypeOptions dspi_CPHA: Data is captured on the leading edge of SCK and changed on the following edge | Data is changed on the leading edge of SCK and captured on the following edge
      mask TypeOptions dspi_LSBFE: MSB first | LSB first
      mask TypeOptions dspi_PCSSCK: 1 | 3 | 5 | 7
      mask TypeOptions dspi_PASC: 1 | 3 | 5 | 7
      mask TypeOptions dspi_PDT: 1 | 3 | 5 | 7
      mask TypeOptions dspi_PBR: 1 | 3 | 5 | 7
      mask TypeOptions dspi_CSSCK: 2 | 4 | 8 | 16 | 32 | 64 | 128 | 256 | 512 | 1024 | 2048 | 4096 | 8192 | 16384 | 32768 | 65536
      mask TypeOptions dspi_ASC: 2 | 4 | 8 | 16 | 32 | 64 | 128 | 256 | 512 | 1024 | 2048 | 4096 | 8192 | 16384 | 32768 | 65536
      mask TypeOptions dspi_DT: 2 | 4 | 8 | 16 | 32 | 64 | 128 | 256 | 512 | 1024 | 2048 | 4096 | 8192 | 16384 | 32768 | 65536
      mask TypeOptions dspi_BR: 2 | 4 | 6 | 8 | 16 | 32 | 64 | 128 | 256 | 512 | 1024 | 2048 | 4096 | 8192 | 16384 | 32768
      mask TypeOptions dspi_PCSIS0: Low | High
      mask TypeOptions dspi_PCSIS1: Low | High
      mask TypeOptions dspi_PCSIS2: Low | High
      mask TypeOptions dspi_PCSIS3: Low | High
      mask TypeOptions dspi_PCSIS4: Low | High
      mask TypeOptions dspi_PCSIS5: Low | High
      mask TypeOptions dspi_PCSIS6: Low | High
      mask TypeOptions dspi_PCSIS7: Low | High
      mask TypeOptions dspi_DIS_RXF: Enable | Disabe | Oops
      mask Callback dspi_DIS_RXF:
      | param = get_param(gcb,'dspi_DIS_RXF');
      | 
      | if (strcmp(param,'Oops') == 0)
      |     if (strcmp(param,'Enable'))
      |         set_param(gcb, 'dspi_DIS_RXF_v2', 'Enable');
      |     else
      |         set_param(gcb, 'dspi_DIS_RXF_v2', 'Disable');
      |     end
      | end
      | 
      | set_param(gcb, 'dspi_DIS_RXF', 'Oops');
      mask Display: disp(st);
  DSPI ISR : S-Function  FunctionName=dspi_564xl_isr  Parameters=dspiInfoOut  EnableBusSupport=off  mask(DSPI_564xL_isr){dspi_Num=0, dspi_isr_name=TCF - Transfer Complete, dspi_isrPrio=14, dspi_isr_tfuf=off, dspi_isr_rfof=on}
      mask prompts: dspi_Num "DSPI"; dspi_isr_name "ISR"; dspi_isrPrio "ISR Priority"; dspi_isr_tfuf "TFUF"; dspi_isr_rfof "RFOF"
      mask help: Read data from a DSPI module.
      mask init:
      | crlf = sprintf('\n');
      | 
      | maskVis = get_param(gcb, 'MaskVisibilities');
      | 
      | dspiNum = get_param(gcb, 'dspi_Num');
      | isr_name = get_param(gcb, 'dspi_isr_name');
      | isr_prio = get_param(gcb, 'dspi_isrPrio');
      | output = 0;
      | [dspiInfoOut,output] = rappid_564xl_dspi_isr_get_info(gcb);
      | 
      | st = ['DSPI: ', dspiNum,crlf,...
      |       'ISR: ', isr_name, crlf,...
      |       'ISR Priority: ', isr_prio];
      mask Help: web([rappid_block_help,filesep,'DSPI_isr.htm']);
      mask TypeOptions dspi_Num: 0 | 1 | 2
      mask TypeOptions dspi_isr_name: Tx/Rx FIFO Underflow/Overflow | EOQF - End of Queue | TFFF - Transmit FIFO Full | TCF - Transfer Complete | RFDF - Rx FIFO Drain
      mask Callback dspi_isr_name:
      | maskVis = get_param(gcb, 'MaskVisibilities');
      | 
      | isr_name = get_param(gcb, 'dspi_isr_name');
      | 
      | maskVis{4} = 'off';
      | maskVis{5} = 'off';
      | 
      | if (strcmp(isr_name,'Tx/Rx FIFO Underflow/Overflow'))
      |     maskVis{4} = 'on';
      |     maskVis{5} = 'on';
      | end
      | 
      | set_param(gcb, 'MaskVisibilities', maskVis);
      mask TypeOptions dspi_isrPrio: 1 | 2 | 3 | 4 | 5 | 6 | 7 | 8 | 9 | 10 | 11 | 12 | 13 | 14 | 15
      mask Display:
      | disp(st);
      | port_label('output', 1, 'trigger')
  DSPI Receive : S-Function  FunctionName=dspi_564xl_receive  Parameters=dspi_Num  EnableBusSupport=off  mask(DSPI_564xL_Receive){dspi_Num=0}
      mask prompts: dspi_Num "DSPI"
      mask help: Read data from a DSPI module.
      mask init:
      | crlf = sprintf('\n');
      | 
      | dspiNum = get_param(gcb, 'dspi_Num');
      | 
      | st = ['DSPI: ', dspiNum];
      mask Help: web([rappid_block_help,filesep,'DSPI_Receive.htm']);
      mask TypeOptions dspi_Num: 0 | 1 | 2
      mask Display:
      | disp(st);
      | port_label('output', 1, 'data')
  DSPI Receive Trigger : S-Function  FunctionName=dspi_564xl_receive_trg  Parameters=dspi_Num  EnableBusSupport=off  mask(DSPI_564xL_Receive_trg){dspi_Num=1, dspi_ISRPri=14}
      mask prompts: dspi_Num "DSPI"; dspi_ISRPri "ISR Priority"
      mask help: Flag to indicate when data is ready to be read from DSPI module.
      mask init:
      | crlf = sprintf('\n');
      | 
      | dspiNum = get_param(gcb, 'dspi_Num');
      | dspiISR = get_param(gcb, 'dspi_ISRPri');
      | 
      | st = ['DSPI: ', dspiNum, crlf,' ISR Priority: ', dspiISR];
      mask Help: web([rappid_block_help,filesep,'DSPI_Receive_trg.htm']);
      mask TypeOptions dspi_Num: 0 | 1 | 2
      mask TypeOptions dspi_ISRPri: 0 | 1 | 2 | 3 | 4 | 5 | 6 | 7 | 8 | 9 | 10 | 11 | 12 | 13 | 14 | 15
      mask Display:
      | disp(st);
      | port_label('output', 1, 'trigger')
      | port_label('output', 2, 'data')
  DSPI Transmit : S-Function  Priority=2  FunctionName=dspi_564xl_transmit  Parameters=dspi_Num, TX_SET, dspiOut  EnableBusSupport=off  mask(DSPI_564xL_Transmit){dspi_Num=0, dspi_CONT=off, dspi_PUSHR_PE=off, dspi_PUSHR_PP=off, dspi_PCS_0=36 : C[4] : [11] : [H3] : CS0, dspi_PCS_1=5 : A[5] : [14] : [H4] : CS0, dspi_PCS_2=3 : A[3] : [92] : [K17] : CS0, dspi_PCS_slave_0=36 : C[4] : [11] : [H3] : CS0, dspi_PCS_slave_1=5 : A[5] : [14] : [H4] : CS0, dspi_PCS_slave_2=3 : A[3] : [92] : [K17] : CS0, dspi_SIN_0=39 : C[7] : [15] : [K4] : SIN, dspi_SIN_1=8 : A[8] : [12] : [F4], dspi_SIN_2=2 : A[2] : [84] : [N16] : SIN, dspi_SCK_0=37 : C[5] : [13] : [G3] : SCK, dspi_SCK_1=6 : A[6] : [2] : [G4] : SCK, dspi_SCK_2=0 : A[0] : [73] : [T14] : SCK, dspi_SOUT_0=38 : C[6] : [142] : [D4] : SOUT, dspi_SOUT_1=7 : A[7] : [10] : [F3] : SOUT, dspi_SOUT_2=1 : A[1] : [74] : [R14] : SOUT, dspi_Strobe=None, dspi_eoq=off, dspi_pcsx=Assert}
      mask prompts: dspi_Num "DSPI"; dspi_CONT "Continuous Peripheral Chip Select Enable"; dspi_PUSHR_PE "Parity Enable"; dspi_PUSHR_PP "Parity Polarity"; dspi_PCS_0 "CS"; dspi_PCS_1 "CS"; dspi_PCS_2 "CS"; dspi_PCS_slave_0 "CS"; dspi_PCS_slave_1 "CS"; dspi_PCS_slave_2 "CS"; dspi_SIN_0 "SIN"; dspi_SIN_1 "SIN"; dspi_SIN_2 "SIN"; dspi_SCK_0 "SCK"; dspi_SCK_1 "SCK"; dspi_SCK_2 "SCK"; dspi_SOUT_0 "SOUT"; dspi_SOUT_1 "SOUT"; dspi_SOUT_2 "SOUT"; dspi_Strobe "CS Strobe"; dspi_eoq "Enable EOQ"; dspi_pcsx "PCSx"
      mask help:
      | Allows to transmit data through a DSPI module.
      | CS Legend (PCR : Port Name : [ Pin# 144pkg ] : [ Pin# 257pkg ])
      mask init:
      | crlf = sprintf('\n');
      | 
      | dspiInfoOut = rappid_564xl_dspi_get_info(gcb);
      | dspiNum = get_param(gcb, 'dspi_Num');
      | dspiMode = rappid_564xl_dspi_get_mode_num(str2num(dspiNum));
      | 
      | 
      | st = ['DSPI: ', dspiNum, crlf, 'CS',dspiInfoOut.csNum,': ', dspiInfoOut.cspinNum,' ', dspiInfoOut.csportName, crlf,...
      |     'SIN: ', dspiInfoOut.sinpinNum,' ', dspiInfoOut.sinportName, crlf,...
      |     'SOUT: ', dspiInfoOut.soutpinNum,' ', dspiInfoOut.soutportName, crlf,...
      |     'SCK: ', dspiInfoOut.sckpinNum,' ', dspiInfoOut.sckportName    
      | ];
      | 
      | dspiNum = str2num(dspiNum);
      | 
      | TX_SET = 0;
      | if ( strcmp(get_param(gcb, 'dspi_CONT'), 'on'))
      |     TX_SET = bitset(uint16(TX_SET), 16);
      | end    
      | if (strcmp(get_param(gcb, 'dspi_PUSHR_PE'), 'on'))
      |     TX_SET = bitset(uint16(TX_SET), 10);
      | end    
      | if ( strcmp(get_param(gcb, 'dspi_PUSHR_PP'), 'on'))
      |     TX_SET = bitset(uint16(TX_SET), 9);
      | end
      | 
      | if (strcmp(get_param(gcb, 'dspi_pcsx'), 'Assert'))
      |     TX_SET = bitset(uint16(TX_SET),str2num(dspiInfoOut.csNum)+1);
      | end
      | 
      | if (strcmp(dspiInfoOut.eoq,'on'))
      |     dspiInfoOut.eoq = 1;
      | else
      |     dspiInfoOut.eoq = 0;
      | end
      | 
      | dspiOut = [str2num(dspiInfoOut.cspcrNum),...
      |     str2num(dspiInfoOut.sinpcrNum),...
      |     str2num(dspiInfoOut.soutpcrNum),...
      |     str2num(dspiInfoOut.sckpcrNum),...
      |     str2num(dspiInfoOut.strobe),...
      |     dspiInfoOut.eoq];
      | 
      | labels = [];
      | str_disp = 'disp(st);';
      | 
      | str_pi1 = 'port_label(''input'',1,''Data'')';
      | str_pi2 = 'port_label(''input'',2,''EOQ'')';
      | 
      | labels = [labels str_pi1 char(10)];
      | if (1 == dspiInfoOut.eoq)
      |     labels = [labels str_pi2 char(10)];
      | end
      | 
      | labels = [labels str_disp char(10)];
      | labels(end) = [];
      | 
      | set_param(gcb,'MaskDisplay',labels);
      mask Help: web([rappid_block_help,filesep,'DSPI_Transmit.htm']);
      mask TypeOptions dspi_Num: 0 | 1 | 2
      mask Callback dspi_Num:
      | param = str2num(get_param(gcb, 'dspi_Num'));
      | MaskVisibilities = get_param(gcb, 'MaskVisibilities');
      | for i=2:22
      |     MaskVisibilities{i} = 'off';
      | end
      | 
      | mode = rappid_564xl_dspi_get_mode_num(param);
      | if (mode == 0)%slave
      |     MaskVisibilities{8+param} = 'on';%cs
      | elseif (mode == 1)%master
      |     MaskVisibilities{5+param} = 'on';%cs
      |     MaskVisibilities{2} = 'on';%cont
      |     MaskVisibilities{3} = 'on';%pe
      |     MaskVisibilities{4} = 'on';%pp
      |     MaskVisibilities{20} = 'on';%strobe
      |     MaskVisibilities{22} = 'on';%pcsx
      | end
      | 
      | MaskVisibilities{21} = 'on';%eoq
      | MaskVisibilities{11+param} = 'on';%sin
      | MaskVisibilities{14+param} = 'on';%sck
      | MaskVisibilities{17+param} = 'on';%sout
      | set_param (gcb,'MaskVisibilities', MaskVisibilities);
      mask TypeOptions dspi_PCS_0: 5 : A[5] : [14] : [H4] : CS7 | 36 : C[4] : [11] : [H3] : CS0 | 53 : D[5] : [33] : [N3] : CS3 | 54 : D[6] : [34] : [P3] : CS2 | 55 : D[7] : [37] : [R4] : CS4 | 56 : D[8] : [32] : [M3] : CS5 | 79 : E[15] : [121] : [B11] : CS1 | 83 : F[3] : [139] : [B5] : CS6 | 104 : G[8] : [81] : [P16] : CS1 | 117 : H[5] : [---] : [M17] : CS4 | 118 : H[6] : [---] : [H17] : CS5 | 120 : H[8] : [---] : [K15] : CS6 | 121 : H[9] : [---] : [G16] : CS7 | 128 : I[0] : [---] : [C9] : CS4 | 129 : I[1] : [---] : [C12] : CS5 | 130 : I[2] : [---] : [F16] : CS6 | 131 : I[3] : [---] : [E17] : CS7
      mask TypeOptions dspi_PCS_1: 5 : A[5] : [14] : [H4] : CS0 | 55 : D[7] : [37] : [R4] : CS3 | 56 : D[8] : [32] : [M3] : CS2 | 98 : G[2] : [102] : [E16] : CS1 | 105 : G[9] : [79] : [R17] : CS1
      mask TypeOptions dspi_PCS_2: 3 : A[3] : [92] : [K17] : CS0 | 4 : A[4] : [108] : [C16] : CS1 | 9 : A[9] : [134] : [B6] : CS1 | 10 : A[10] : [118] : [A13] : CS0 | 22 : B[6] : [138] : B[3] : CS2 | 42 : C[10] : [111] : [A15] : CS2 | 43 : C[11] : [80] : [M14] : CS2 | 44 : C[12] : [82] : [N15] : CS3 | 77: E[13] : [117] : [D12] : CS3 | 101: G[5] : [85] : [N17] : CS3 | 106: G[10] : [77] : [P15] : CS3
      mask TypeOptions dspi_PCS_slave_0: 36 : C[4] : [11] : [H3] : CS0
      mask TypeOptions dspi_PCS_slave_1: 5 : A[5] : [14] : [H4] : CS0
      mask TypeOptions dspi_PCS_slave_2: 3 : A[3] : [92] : [K17] : CS0 | 10 : A[10] : [118] : [A13] : CS0
      mask TypeOptions dspi_SIN_0: 39 : C[7] : [15] : [K4] : SIN
      mask TypeOptions dspi_SIN_1: 8 : A[8] : [12] : [F4]
      mask TypeOptions dspi_SIN_2: 2 : A[2] : [84] : [N16] : SIN | 13: A[13] : [136] : [C6] : SIN
      mask TypeOptions dspi_SCK_0: 37 : C[5] : [13] : [G3] : SCK
      mask TypeOptions dspi_SCK_1: 6 : A[6] : [2] : [G4] : SCK
      mask TypeOptions dspi_SCK_2: 0 : A[0] : [73] : [T14] : SCK | 11 : A[11] : [120] : [D11] : SCK
      mask TypeOptions dspi_SOUT_0: 38 : C[6] : [142] : [D4] : SOUT
      mask TypeOptions dspi_SOUT_1: 7 : A[7] : [10] : [F3] : SOUT
      mask TypeOptions dspi_SOUT_2: 1 : A[1] : [74] : [R14] : SOUT | 12 : A[12] : [122] : [A10] : SOUT
      mask TypeOptions dspi_Strobe: None | 56 : D[8] : [32] : [M3] : CS5 | 118 : H[6] : [---] : [H17] : CS5 | 129 : I[1] : [---] : [C12] : CS5
      mask TypeOptions dspi_pcsx: Negate | Assert
      mask Display:
      | port_label('input',1,'Data')
      | disp(st);
  DSPI interrupt enable-disable : S-Function  FunctionName=dspi_564xl_disable_isr  Parameters=dspiInfoOut  EnableBusSupport=off  mask(dspi_564xl_isr_enable){dspi_Num=0, dspi_isr_tfuf=off, dspi_isr_rfof=off, EOQF_enable=off, TFFF_enable=off, TCF_enable=off, RFDF_enable=off}
      mask prompts: dspi_Num "DSPI"; dspi_isr_tfuf "Enable TFUF"; dspi_isr_rfof "Enable RFOF"; EOQF_enable "Enable EOQF - End of Queue"; TFFF_enable "Enable TFFF - Transmit FIFO Full"; TCF_enable "Enable TCF - Transfer Complete"; RFDF_enable "Enable RFDF - Rx FIFO Drain"
      mask help: This block enables or disables the interrupt for each DSPI block.
      mask init:
      | crlf = sprintf('\n');
      | 
      | dspiNum = get_param(gcb, 'dspi_Num');
      | 
      | tx_str   =  get_param(gcb, 'dspi_isr_tfuf');
      | rx_str   =  get_param(gcb, 'dspi_isr_rfof');
      | EOQF_str =  get_param(gcb, 'EOQF_enable');
      | TFFF_str =  get_param(gcb, 'TFFF_enable');
      | TCF_str  =  get_param(gcb, 'TCF_enable');
      | RFDF_str  =  get_param(gcb, 'RFDF_enable');
      | 
      | dspi_st = 0;
      | if strcmp(tx_str, 'on')
      |     dspi_st = bitset(uint16(dspi_st),1);
      | end
      | if strcmp(rx_str, 'on')
      |     dspi_st = bitset(uint16(dspi_st),2);
      | end
      | if strcmp(EOQF_str, 'on')
      |     dspi_st = bitset(uint16(dspi_st),3);
      | end
      | if strcmp(TFFF_str, 'on')
      |     dspi_st = bitset(uint16(dspi_st),4);
      | end
      | if strcmp(RFDF_str, 'on')
      |     dspi_st = bitset(uint16(dspi_st),6);
      | end
      | if strcmp(TCF_str, 'on')
      |     dspi_st = bitset(uint16(dspi_st),5);
      | end
      | 
      | dspiNum_dig = str2num(dspiNum);
      | dspiInfoOut = [dspiNum_dig, dspi_st];
      | 
      | st = ['DSPI: ', dspiNum, crlf, 'Enable interrupt: ', dec2bin(dspi_st,8)];
      mask Help: web([rappid_block_help,filesep,'DSPI_isr_enable.htm']);
      mask TypeOptions dspi_Num: 0 | 1 | 2
      mask Display: disp(st);
